simulink model "Problem_2"  (R2020b)
settings: Solver=VariableStepAuto  StartTime=0.0  StopTime=500  RelTol=1e-3
values from neighbouring files (symbols this model uses):
  B1 = 50    [p.m]
  B2 = 25    [p.m]
  K1 = 50    [p.m]
  K2 = 50    [p.m]
  M1 = 100    [p.m]
  M2 = 50    [p.m]
settings Model: Creator=HP  LastModifiedBy=HP

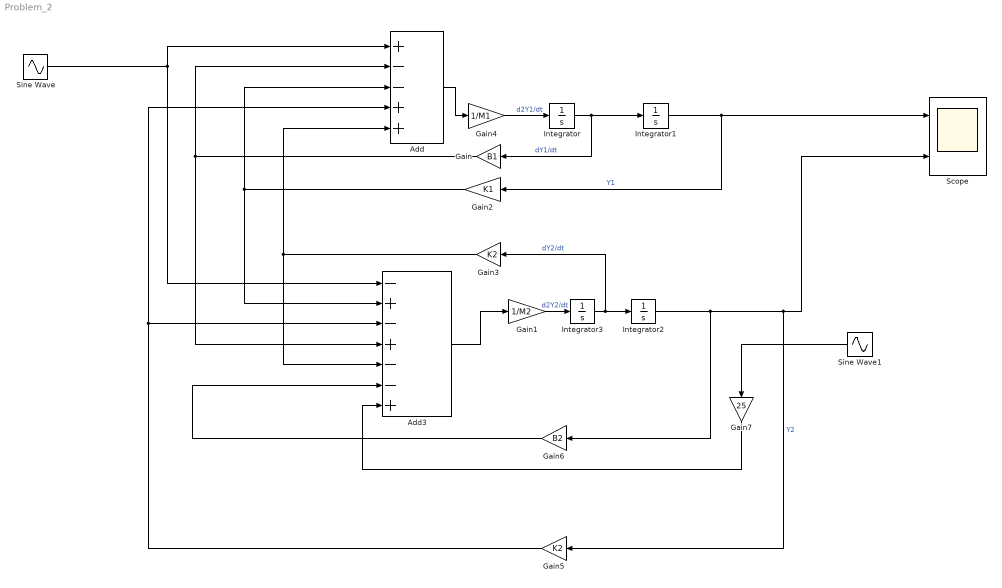
== system Problem_2 ==
  Add : Sum  Inputs=+--++
  Add3 : Sum  Inputs=-+-+--+
  Gain : Gain  Gain=B1
  Gain1 : Gain  Gain=1/M2
  Gain2 : Gain  Gain=K1
  Gain3 : Gain  Gain=K2
  Gain4 : Gain  Gain=1/M1
  Gain5 : Gain  Gain=K2
  Gain6 : Gain  Gain=B2
  Gain7 : Gain  Gain=25
  Integrator{,1..3} (4 alike) : Integrator
  Scope : Scope  NumInputPorts=2
  Sine Wave : Sin  Amplitude=2  Frequency=10  SampleTime=0
  Sine Wave1 : Sin  Amplitude=2  Frequency=10  SampleTime=0
  wires:
  Sine Wave1/1 -> Gain7/1
  Sine Wave/1 -> Add/1, Add3/1
  Gain/1 -> Add3/4, Add/2
  Integrator3/1 -> Gain3/1, Integrator2/1  "dY2/dt"
  Gain6/1 -> Add3/6
  Add/1 -> Gain4/1
  Gain3/1 -> Add3/5, Add/5
  Gain5/1 -> Add/4, Add3/3
  Add3/1 -> Gain1/1
  Gain2/1 -> Add3/2, Add/3
  Gain7/1 -> Add3/7
  Gain1/1 -> Integrator3/1  "d2Y2/dt"
  Integrator2/1 -> Gain6/1, Scope/2, Gain5/1  "Y2"
  Gain4/1 -> Integrator/1  "d2Y1/dt"
  Integrator1/1 -> Gain2/1, Scope/1  "Y1"
  Integrator/1 -> Gain/1, Integrator1/1  "dY1/dt"
